simulink model "LQR"  (R2021a)
settings: Solver=VariableStepAuto  StartTime=0.0  StopTime=2  RelTol=1e-3
values from neighbouring files (symbols this model uses):
  A = [1  0; 2  0]    [LQR.mat]
  B = [1 0]    [LQR.mat]
  C = [0 1]    [LQR.mat]
  K = [12.2911959688 31.6227766017]    [LQR.mat]
  Mbar = 31.6227766017    [LQR.mat]
settings Model: Creator=Admin  LastModifiedBy=Admin

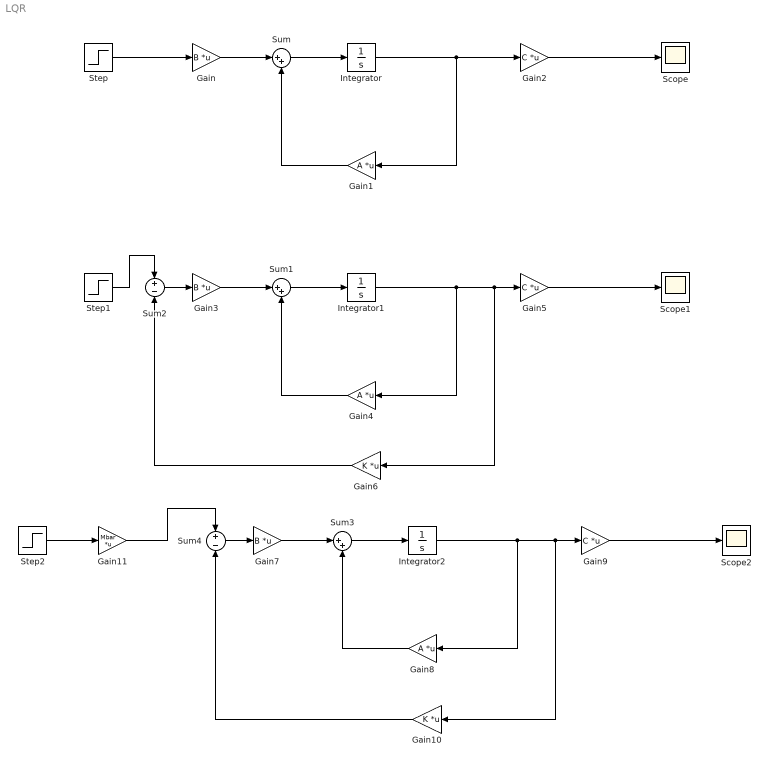
== system LQR ==
  Gain : Gain  Gain=B  Multiplication=Matrix(K*u)
  Gain1 : Gain  Gain=A  Multiplication=Matrix(K*u)
  Gain10 : Gain  Gain=K  Multiplication=Matrix(K*u)
  Gain11 : Gain  Gain=Mbar  Multiplication=Matrix(K*u)
  Gain2 : Gain  Gain=C  Multiplication=Matrix(K*u)
  Gain3 : Gain  Gain=B  Multiplication=Matrix(K*u)
  Gain4 : Gain  Gain=A  Multiplication=Matrix(K*u)
  Gain5 : Gain  Gain=C  Multiplication=Matrix(K*u)
  Gain6 : Gain  Gain=K  Multiplication=Matrix(K*u)
  Gain7 : Gain  Gain=B  Multiplication=Matrix(K*u)
  Gain8 : Gain  Gain=A  Multiplication=Matrix(K*u)
  Gain9 : Gain  Gain=C  Multiplication=Matrix(K*u)
  Integrator : Integrator
  Integrator1 : Integrator
  Integrator2 : Integrator
  Scope : Scope
  Scope1 : Scope
  Scope2 : Scope
  Step : Step  SampleTime=0
  Step1 : Step  Time=0  SampleTime=0
  Step2 : Step  Time=0  SampleTime=0
  Sum : Sum  Inputs=|++
  Sum1 : Sum  Inputs=|++
  Sum2 : Sum  Inputs=+-
  Sum3 : Sum  Inputs=|++
  Sum4 : Sum  Inputs=+-
  wires:
  Gain1/1 -> Sum/2
  Gain/1 -> Sum/1
  Sum/1 -> Integrator/1
  Integrator/1 -> Gain1/1, Gain2/1
  Gain2/1 -> Scope/1
  Step/1 -> Gain/1
  Sum1/1 -> Integrator1/1
  Integrator1/1 -> Gain4/1, Gain6/1, Gain5/1
  Gain5/1 -> Scope1/1
  Gain3/1 -> Sum1/1
  Gain4/1 -> Sum1/2
  Step1/1 -> Sum2/1
  Sum2/1 -> Gain3/1
  Gain6/1 -> Sum2/2
  Gain10/1 -> Sum4/2
  Gain9/1 -> Scope2/1
  Gain8/1 -> Sum3/2
  Integrator2/1 -> Gain8/1, Gain10/1, Gain9/1
  Gain7/1 -> Sum3/1
  Sum4/1 -> Gain7/1
  Sum3/1 -> Integrator2/1
  Step2/1 -> Gain11/1
  Gain11/1 -> Sum4/1
